simulink model "p1_rc_sim"  (R2024a)
settings: Solver=VariableStepAuto  StartTime=0.0  StopTime=0.1  MaxStep=50e-6  RelTol=1e-3
values from neighbouring files (symbols this model uses):
  C = 470e-9    (= 4.7e-07)    [p1_rc_ini.m]
  R = 4.7e3    (= 4700)    [p1_rc_ini.m]
settings Model: Creator=PMIC  LastModifiedBy=miche
settings DataIOCC: SaveOutput=off  SignalLogging=off  DSMLogging=off  SaveTime=off  ReturnWorkspaceOutputs=off
settings RTWCC: GPUComputeCapability=3.5

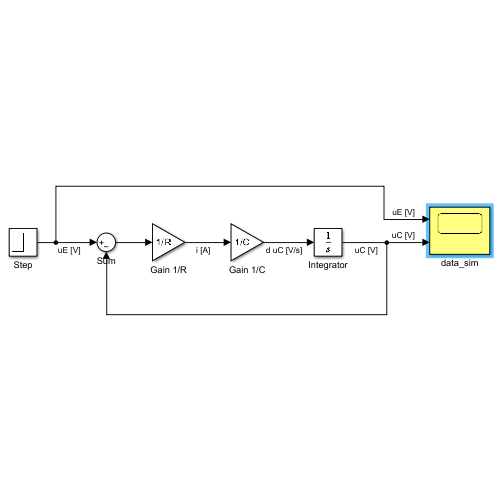
[thumbnail: Simulink's stored preview of the top-level diagram]
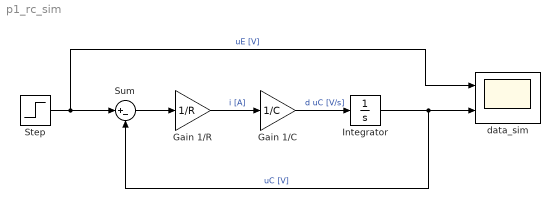
== system p1_rc_sim ==
  Gain 1/C : Gain  Gain=1/C
  Gain 1/R : Gain  Gain=1/R
  Integrator : Integrator
  Step : Step  Time=0.05  SampleTime=0
  Sum : Sum  Inputs=|+-
  data_sim : Scope  NumInputPorts=2
      settings: CopyFcn=try ZHAWcbfcn('copyScope'); end  NameChangeFcn=try ZHAWcbfcn('namechangeScope'); end
  wires:
  Integrator/1 -> data_sim/2, Sum/2  "uC [V]"
  Step/1 -> data_sim/1, Sum/1  "uE [V]"
  Sum/1 -> Gain 1/R/1
  Gain 1/R/1 -> Gain 1/C/1  "i [A]"
  Gain 1/C/1 -> Integrator/1  "d uC [V/s]"
